simulink model "LQT_Simulation"  (R2015b)
settings: Solver=FixedStepAuto  StartTime=0.0  StopTime=tsim  FixedStep=Ts  RelTol=1e-3
values from neighbouring files (symbols this model uses):
  A_kal = [1 0 0 Ts 0 0 ... (first row only)    [LQT_12states.m]
  C_kal = [1 0 0 0 0 0 ... (first row only)    [LQT_12states.m]
  Ki = [-Ki_coef_ang  -Ki_coef_ang   -Ki_coef_ang ... (first row only)    [LQT_12states.m]
  Ki_LQT = [Ki_coef  -Ki_coef   -Ki_coefz ... (first row only)    [LQT_12states.m]
  R_kal = diag([5e-9 5e-9 5e-9])    [LQT_12states.m]
  Ts = 0.01    [LQT_12states.m]    (also in Trajectory_generation.m)
  VAR_XY = 5e-9    (= 5e-09)    [LQT_12states.m]
  VAR_Z = 5e-9    (= 5e-09)    [LQT_12states.m]
undefined symbols (not defined in the file or in its folder): DiscIntNeverNeededParam, Discrete, pwm, quad, Time
libraries: realtime_pacer_lib x2, ctrlSharedLib x1, aerolibtransform2 x1
settings Model: SimulationMode=accelerator  Creator=carlosluis  LastModifiedBy=carlosluis
settings DebuggingCC: MultiTaskRateTransMsg=warning

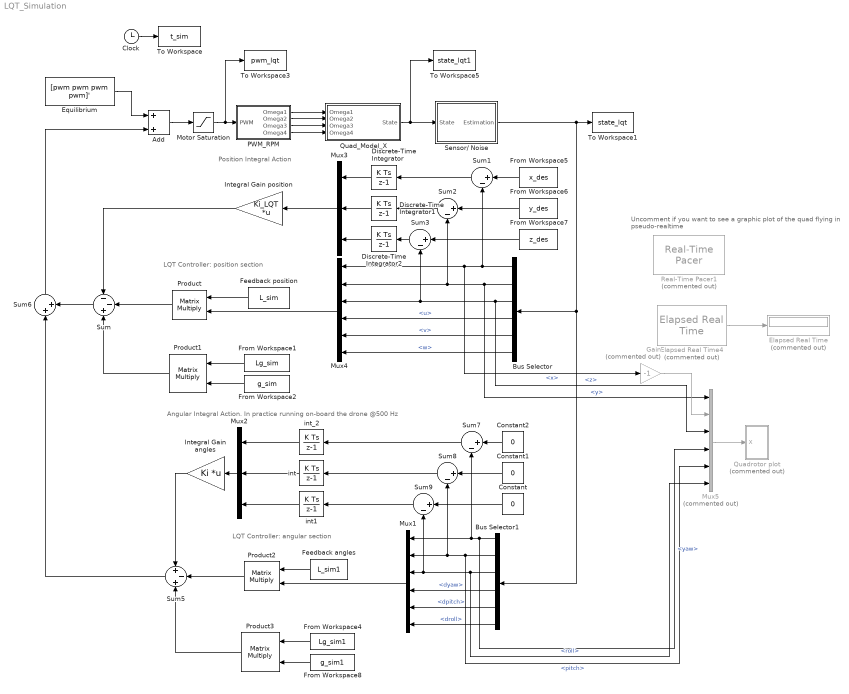
== system LQT_Simulation ==
  note: Uncomment if you want to see a graphic plot of the quad
      | flying in pseudo-realtime
  note: Position Integral Action
  note: Angular Integral Action. In practice running on-board the drone @500 Hz
  note: LQT Controller: position section
  note: LQT Controller: angular section
  Add : Sum
  Bus Selector : BusSelector  OutputSignals=signal1.x,signal1.y,signal1.z,signal3.u,signal3.v,signal3.w
  Bus Selector1 : BusSelector  OutputSignals=signal2.yaw,signal2.pitch,signal2.roll,signal4.dyaw,signal4.dpitch,signal4.droll
  Clock : Clock
  Constant : Constant  Value=0
  Constant1 : Constant  Value=0
  Constant2 : Constant  Value=0
  Discrete-Time Integrator : DiscreteIntegrator  gainval=1  InitialConditionSetting=State (most efficient)  SampleTime=Ts  ICPrevOutput=DiscIntNeverNeededParam  ICPrevScaledInput=DiscIntNeverNeededParam
  Discrete-Time Integrator1 : DiscreteIntegrator  gainval=1  InitialConditionSetting=State (most efficient)  SampleTime=Ts  ICPrevOutput=DiscIntNeverNeededParam  ICPrevScaledInput=DiscIntNeverNeededParam
  Discrete-Time Integrator2 : DiscreteIntegrator  gainval=1  InitialConditionSetting=State (most efficient)  SampleTime=Ts  ICPrevOutput=DiscIntNeverNeededParam  ICPrevScaledInput=DiscIntNeverNeededParam
  Elapsed Real Time : Display  Commented=on
      settings: Decimation=2
  Elapsed Real Time4 : realtime_pacer_lib/Elapsed Real Time  Commented=on
  Equilibrium : Constant  Value=[pwm pwm pwm pwm]'
  Feedback angles : FromWorkspace  VariableName=L_sim1  SampleTime=Ts
  Feedback position : FromWorkspace  VariableName=L_sim  SampleTime=Ts
  From Workspace1 : FromWorkspace  VariableName=Lg_sim  SampleTime=Ts
  From Workspace2 : FromWorkspace  VariableName=g_sim  SampleTime=Ts
  From Workspace4 : FromWorkspace  VariableName=Lg_sim1  SampleTime=Ts
  From Workspace5 : FromWorkspace  VariableName=x_des  SampleTime=Ts
  From Workspace6 : FromWorkspace  VariableName=y_des  SampleTime=Ts
  From Workspace7 : FromWorkspace  VariableName=z_des  SampleTime=Ts
  From Workspace8 : FromWorkspace  VariableName=g_sim1  SampleTime=Ts
  Gain : Gain  Commented=on  Gain=-1
  Integral Gain angles : Gain  Gain=Ki  Multiplication=Matrix(K*u)
  Integral Gain position : Gain  Gain=Ki_LQT  Multiplication=Matrix(K*u)
  Motor Saturation : Saturate  UpperLimit=60000
  Mux1 : Mux  Inputs=6
  Mux2 : Mux  Inputs=3
  Mux3 : Mux  Inputs=3
  Mux4 : Mux  Inputs=6
  Mux5 : Mux  Commented=on  Inputs=6
  PWM_RPM : Subsystem
  Product{,1..3} (4 alike) : Product  Multiplication=Matrix(*)
  Quad_Model_X : Subsystem
  Quadrotor plot : Subsystem  Commented=on  AncestorBlock=roblocks/Robot Graphics/Quadrotor plot  mask{quad=quad, xydim=2, zdim=2.3}
      mask prompts: quad "Model"; xydim "xy-axes dimension"; zdim "z-axis dimension"
      mask help: Animate quadrotor.
      mask Help:
      | This block graphically displays a quadrotor (flying robot).
      | 
      | A new figure is created and A graphical model of a quadrotor is animated
      | to a pose specified by the state vector input to the block.
      | 
      | The state vector is [x y z roll pitch yaw] in world coordinates and the
      | angles are in radians.
      | 
      | Notes:
      | - The dimensions of the vehicle workspace are set by parameters
  Real-Time Pacer1 : realtime_pacer_lib/Real-Time Pacer  Commented=on  simTimePerRealTime=1
  Sensor/ Noise : Subsystem
  Sum : Sum  Inputs=--+
  Sum{1..3,7..9} (6 alike) : Sum  Inputs=|+-
  Sum5 : Sum  Inputs=+-+
  Sum6 : Sum  Inputs=|++
  To Workspace : ToWorkspace  VariableName=t_sim  SampleTime=Ts
  To Workspace1 : ToWorkspace  VariableName=state_lqt  SampleTime=Ts
  To Workspace3 : ToWorkspace  VariableName=pwm_lqt  SampleTime=Ts
  To Workspace5 : ToWorkspace  VariableName=state_lqt1  SampleTime=Ts
  int : DiscreteIntegrator  gainval=1  InitialConditionSetting=State (most efficient)  SampleTime=Ts  ICPrevOutput=DiscIntNeverNeededParam  ICPrevScaledInput=DiscIntNeverNeededParam
  int1 : DiscreteIntegrator  gainval=1  InitialConditionSetting=State (most efficient)  SampleTime=Ts  ICPrevOutput=DiscIntNeverNeededParam  ICPrevScaledInput=DiscIntNeverNeededParam
  int_2 : DiscreteIntegrator  gainval=1  InitialConditionSetting=State (most efficient)  SampleTime=Ts  ICPrevOutput=DiscIntNeverNeededParam  ICPrevScaledInput=DiscIntNeverNeededParam
  wires:
  From Workspace1/1 -> Product1/1
  From Workspace2/1 -> Product1/2
  Feedback position/1 -> Product/1
  Clock/1 -> To Workspace/1
  PWM_RPM/1(Omega1) -> Quad_Model_X/1(Omega1)
  PWM_RPM/2(Omega2) -> Quad_Model_X/2(Omega2)
  PWM_RPM/3(Omega3) -> Quad_Model_X/3(Omega3)
  PWM_RPM/4(Omega4) -> Quad_Model_X/4(Omega4)
  Add/1 -> Motor Saturation/1
  Motor Saturation/1 -> PWM_RPM/1(PWM), To Workspace3/1
  Quad_Model_X/1(State) -> Sensor/ Noise/1(State), To Workspace5/1
  Sensor/ Noise/1(Estimation) -> Bus Selector/1, Bus Selector1/1, To Workspace1/1
  Sum1/1 -> Discrete-Time Integrator/1
  Sum2/1 -> Discrete-Time Integrator1/1
  Sum3/1 -> Discrete-Time Integrator2/1
  Bus Selector1/1 -> Mux5/4, Mux1/1, Sum7/2  "<yaw>"
  Bus Selector1/2 -> Mux5/5, Sum8/2, Mux1/2  "<pitch>"
  Bus Selector1/3 -> Mux5/6, Sum9/2, Mux1/3  "<roll>"
  Bus Selector1/4 -> Mux1/4  "<dyaw>"
  Bus Selector1/5 -> Mux1/5  "<dpitch>"
  Bus Selector1/6 -> Mux1/6  "<droll>"
  From Workspace4/1 -> Product3/1
  From Workspace8/1 -> Product3/2
  Feedback angles/1 -> Product2/1
  Mux1/1 -> Product2/2
  Sum5/1 -> Sum6/1
  int_2/1 -> Mux2/1
  Sum7/1 -> int_2/1
  int/1 -> Mux2/2
  Sum8/1 -> int/1
  Sum9/1 -> int1/1
  int1/1 -> Mux2/3
  Discrete-Time Integrator/1 -> Mux3/1
  Discrete-Time Integrator1/1 -> Mux3/2
  Discrete-Time Integrator2/1 -> Mux3/3
  Mux3/1 -> Integral Gain position/1
  Product3/1 -> Sum5/3
  Product2/1 -> Sum5/2
  Constant/1 -> Sum9/1
  Constant2/1 -> Sum7/1
  Constant1/1 -> Sum8/1
  Mux2/1 -> Integral Gain angles/1
  Integral Gain angles/1 -> Sum5/1
  From Workspace5/1 -> Sum1/1
  From Workspace6/1 -> Sum2/1
  From Workspace7/1 -> Sum3/1
  Bus Selector/1 -> Gain/1, Mux4/1, Sum1/2  "<x>"
  Bus Selector/2 -> Mux5/1, Sum2/2, Mux4/2  "<y>"
  Bus Selector/3 -> Mux5/3, Sum3/2, Mux4/3  "<z>"
  Bus Selector/4 -> Mux4/4  "<u>"
  Bus Selector/5 -> Mux4/5  "<v>"
  Bus Selector/6 -> Mux4/6  "<w>"
  Mux4/1 -> Product/2
  Product1/1 -> Sum/3
  Product/1 -> Sum/2
  Integral Gain position/1 -> Sum/1
  Sum/1 -> Sum6/2
  Sum6/1 -> Add/2
  Equilibrium/1 -> Add/1
  Elapsed Real Time4/1 -> Elapsed Real Time/1
  Mux5/1 -> Quadrotor plot/1(X)
  Gain/1 -> Mux5/2

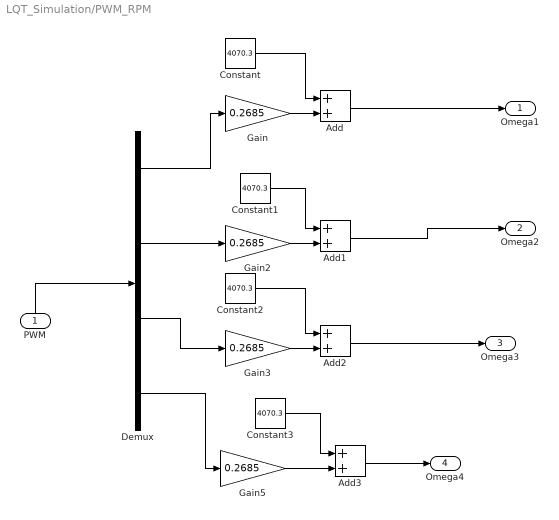
== system LQT_Simulation/PWM_RPM ==
  PWM : Inport
  Add{,1..3} (4 alike) : Sum
  Constant{,1..3} (4 alike) : Constant  Value=4070.3
  Demux : Demux
  Gain{,2..3,5} (4 alike) : Gain  Gain=0.2685
  Omega1 : Outport
  Omega2 : Outport  Port=2
  Omega3 : Outport  Port=3
  Omega4 : Outport  Port=4
  wires:
  Gain/1 -> Add/2
  Demux/1 -> Gain/1
  Demux/4 -> Gain5/1
  Gain5/1 -> Add3/2
  Constant3/1 -> Add3/1
  Add3/1 -> Omega4/1
  Constant1/1 -> Add1/1
  Gain2/1 -> Add1/2
  Demux/2 -> Gain2/1
  Add1/1 -> Omega2/1
  PWM/1 -> Demux/1
  Add/1 -> Omega1/1
  Add2/1 -> Omega3/1
  Demux/3 -> Gain3/1
  Constant2/1 -> Add2/1
  Gain3/1 -> Add2/2
  Constant/1 -> Add/1

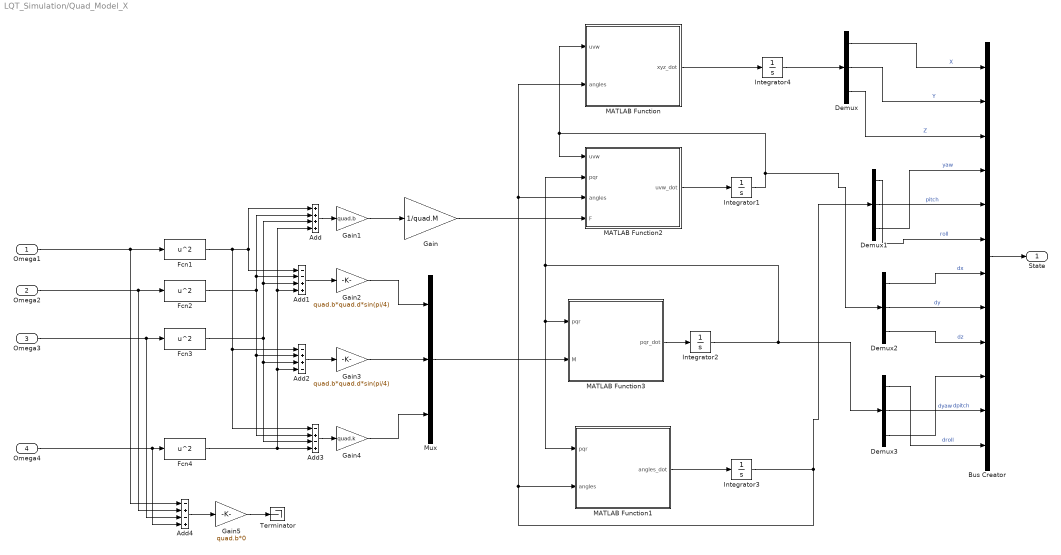
== system LQT_Simulation/Quad_Model_X ==
  Omega1 : Inport
  Omega2 : Inport  Port=2
  Omega3 : Inport  Port=3
  Omega4 : Inport  Port=4
  Add : Sum  Inputs=++++
  Add1 : Sum  Inputs=--++
  Add2 : Sum  Inputs=-++-
  Add3 : Sum  Inputs=-+-+
  Add4 : Sum  Inputs=-+-+
  Bus Creator : BusCreator  Inputs=12
  Demux{,1..3} (4 alike) : Demux  Outputs=3
  Fcn{1..4} (4 alike) : Fcn  Expr=u^2
  Gain : Gain  Gain=1/quad.M
  Gain1 : Gain  Gain=quad.b
  Gain2 : Gain  Gain=quad.b*quad.d*sin(pi/4)
  Gain3 : Gain  Gain=quad.b*quad.d*sin(pi/4)
  Gain4 : Gain  Gain=quad.k
  Gain5 : Gain  Gain=quad.b*0
  Integrator1 : Integrator
  Integrator2 : Integrator
  Integrator3 : Integrator  InitialCondition=[0;0;0]
  Integrator4 : Integrator  InitialCondition=[0;0;0]
  MATLAB Function : MATLAB Function  TreatAsAtomicUnit=on
  MATLAB Function1 : MATLAB Function  TreatAsAtomicUnit=on
  MATLAB Function2 : MATLAB Function  TreatAsAtomicUnit=on
  MATLAB Function3 : MATLAB Function  TreatAsAtomicUnit=on
  Mux : Mux  Inputs=3
  Terminator : Terminator
  State : Outport
  wires:
  Gain1/1 -> Gain/1
  Fcn4/1 -> Add/4, Add1/4, Add2/4, Add3/4
  Fcn3/1 -> Add1/3, Add/3, Add2/3, Add3/3
  Fcn2/1 -> Add2/2, Add3/2, Add1/2, Add/2
  Fcn1/1 -> Add/1, Add1/1, Add2/1, Add3/1
  Bus Creator/1 -> State/1
  Add1/1 -> Gain2/1
  Add/1 -> Gain1/1
  Omega2/1 -> Add4/2, Fcn2/1
  Omega1/1 -> Fcn1/1, Add4/1
  Add2/1 -> Gain3/1
  Gain2/1 -> Mux/1
  Gain4/1 -> Mux/3
  Omega3/1 -> Add4/3, Fcn3/1
  Omega4/1 -> Fcn4/1, Add4/4
  Add4/1 -> Gain5/1
  Add3/1 -> Gain4/1
  Gain3/1 -> Mux/2
  Gain/1 -> MATLAB Function2/4(F)
  Mux/1 -> MATLAB Function3/2(M)
  MATLAB Function2/1(uvw_dot) -> Integrator1/1
  MATLAB Function3/1(pqr_dot) -> Integrator2/1
  MATLAB Function1/1(angles_dot) -> Integrator3/1
  Integrator1/1 -> MATLAB Function/1(uvw), MATLAB Function2/1(uvw), Demux2/1
  Integrator2/1 -> Demux3/1, MATLAB Function2/2(pqr), MATLAB Function1/1(pqr), MATLAB Function3/1(pqr)
  Demux/1 -> Bus Creator/1  "X"
  Demux/2 -> Bus Creator/2  "Y"
  Demux/3 -> Bus Creator/3  "Z"
  Demux1/3 -> Bus Creator/4  "yaw"
  Demux1/1 -> Bus Creator/6  "roll"
  Demux2/1 -> Bus Creator/7  "dx"
  Demux2/2 -> Bus Creator/8  "dy"
  Demux2/3 -> Bus Creator/9  "dz"
  Demux3/3 -> Bus Creator/10  "dyaw"
  Demux3/2 -> Bus Creator/11  "dpitch"
  Demux3/1 -> Bus Creator/12  "droll"
  Gain5/1 -> Terminator/1
  Demux1/2 -> Bus Creator/5  "pitch"
  Integrator3/1 -> Demux1/1, MATLAB Function/2(angles), MATLAB Function2/3(angles), MATLAB Function1/2(angles)
  MATLAB Function/1(xyz_dot) -> Integrator4/1
  Integrator4/1 -> Demux/1

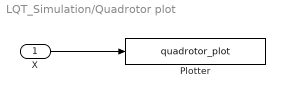
== system LQT_Simulation/Quadrotor plot ==
  X : Inport
  Plotter : S-Function  FunctionName=quadrotor_plot  Parameters=[xydim, zdim], 1, 1,quad  SFunctionDeploymentMode=off  EnableBusSupport=off
  wires:
  X/1 -> Plotter/1

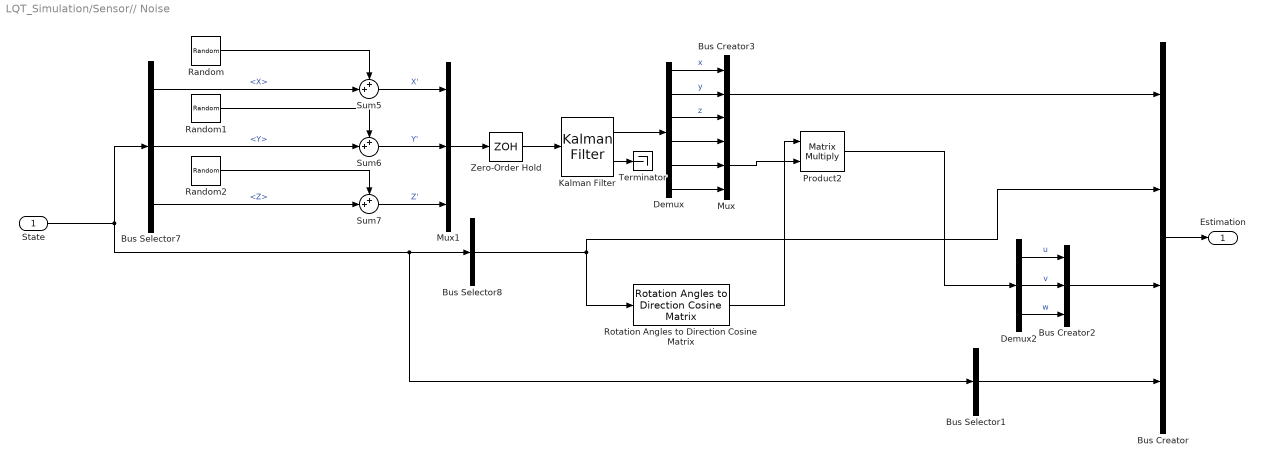
== system LQT_Simulation/Sensor// Noise ==
  State : Inport
  Bus Creator : BusCreator  Inputs=4
  Bus Creator2 : BusCreator  Inputs=3
  Bus Creator3 : BusCreator  Inputs=3
  Bus Selector1 : BusSelector  OutputSignals=dyaw,dpitch,droll  OutputAsBus=on
  Bus Selector7 : BusSelector  OutputSignals=X,Y,Z
  Bus Selector8 : BusSelector  OutputSignals=yaw,pitch,roll  OutputAsBus=on
  Demux : Demux  Outputs=6
  Demux2 : Demux  Outputs=3
  Kalman Filter : ctrlSharedLib/Kalman Filter  TimeDomain=Discrete-Time  UseCurrentEstimator=on  ModelSource=Individual A, B, C, D matrices  ModelSourceVariable=ss(0.95,1,1,0,1)  A=A_kal  B=1  C=C_kal  D=0  NumberOfStates=1  NumberOfInputs=1  NumberOfOutputs=1  InitialEstimateSource=Dialog  X0=0  P0=10  UseK=off  UseGH=on  NumberOfProcessNoiseInputs=1  G=G_kal  TimeInvariantG=on  H=0  TimeInvariantH=on  Q=Q_kal  TimeInvariantQ=on  R=R_kal  TimeInvariantR=on  N=0  TimeInvariantN=on  AddInputPort=off  AddEnablePort=off  OutputEstimatedY=off  OutputP=on  Ts=Ts
  Mux : Mux  Inputs=3
  Mux1 : Mux  Inputs=3
  Product2 : Product  Multiplication=Matrix(*)
  Random : RandomNumber  Variance=VAR_XY  SampleTime=Ts
  Random1 : RandomNumber  Variance=VAR_XY  SampleTime=Ts
  Random2 : RandomNumber  Variance=VAR_Z  SampleTime=Ts
  Rotation Angles to Direction Cosine Matrix : aerolibtransform2/Rotation Angles to Direction Cosine Matrix  rotationOrder=ZYX
  Sum5 : Sum  Inputs=++|
  Sum6 : Sum  Inputs=++|
  Sum7 : Sum  Inputs=++|
  Terminator : Terminator
  Zero-Order Hold : ZeroOrderHold  SampleTime=Ts
  Estimation : Outport
  wires:
  Bus Selector8/1 -> Bus Creator/2, Rotation Angles to Direction Cosine Matrix/1
  Product2/1 -> Demux2/1
  Rotation Angles to Direction Cosine Matrix/1 -> Product2/1
  Kalman Filter/1 -> Demux/1
  Zero-Order Hold/1 -> Kalman Filter/1
  Mux1/1 -> Zero-Order Hold/1
  Bus Creator3/1 -> Bus Creator/1
  Demux/3 -> Bus Creator3/3  "z"
  Demux/2 -> Bus Creator3/2  "y"
  Demux/1 -> Bus Creator3/1  "x"
  Mux/1 -> Product2/2
  Demux/4 -> Mux/1
  Demux/5 -> Mux/2
  Demux/6 -> Mux/3
  Bus Creator2/1 -> Bus Creator/3
  Bus Selector1/1 -> Bus Creator/4
  Demux2/3 -> Bus Creator2/3  "w"
  Demux2/2 -> Bus Creator2/2  "v"
  Demux2/1 -> Bus Creator2/1  "u"
  Random2/1 -> Sum7/1
  Sum7/1 -> Mux1/3  "Z'"
  Sum6/1 -> Mux1/2  "Y'"
  Sum5/1 -> Mux1/1  "X'"
  Bus Selector7/3 -> Sum7/2  "<Z>"
  Bus Selector7/2 -> Sum6/2  "<Y>"
  Bus Selector7/1 -> Sum5/2  "<X>"
  Bus Creator/1 -> Estimation/1
  State/1 -> Bus Selector7/1, Bus Selector1/1, Bus Selector8/1
  Random1/1 -> Sum6/1
  Random/1 -> Sum5/1
  Kalman Filter/2 -> Terminator/1

== matlab function LQT_Simulation/Quad_Model_X/MATLAB Function ==
  data: uvw input; xyz_dot output; angles input
function xyz_dot  = Position(uvw,angles)
xyz_dot = zeros(3,1);
phi = angles(1); %*pi/180;
theta = angles(2); %*pi/180;
psi = angles(3); %*pi/180;
Tb_o = [cos(theta)*cos(psi)                                cos(theta)*sin(psi)                             -sin(theta)  ;   %BBF > Inertial rotation matrix
        sin(phi)*sin(theta)*cos(psi)-cos(phi)*sin(psi)    sin(phi)*sin(theta)*sin(psi)+cos(phi)*cos(psi)  sin(phi)*cos(theta) ;
        cos(phi)*sin(theta)*cos(psi)+sin(phi)*sin(psi)    cos(phi)*sin(theta)*sin(psi)-sin(phi)*cos(psi)   cos(phi)*cos(theta)];

xyz_dot = (Tb_o')*uvw;
end

== matlab function LQT_Simulation/Quad_Model_X/MATLAB Function1 ==
  data: pqr input; angles_dot output; angles input
function angles_dot  = Angle(pqr,angles)
angles_dot = zeros(3,1);
phi = angles(1); %*pi/180;
theta = angles(2); %*pi/180;

H = [1    sin(phi)*tan(theta)     cos(phi)*tan(theta)
     0       cos(phi)                 -sin(phi)   
     0       sin(phi)/cos(theta)    cos(phi)/cos(theta)];
angles_dot = H*pqr;
end

== matlab function LQT_Simulation/Quad_Model_X/MATLAB Function2 ==
  data: uvw input; uvw_dot output; pqr input; angles input; F input
function uvw_dot  = Forces(uvw,pqr,angles,F)
uvw_dot = zeros(3,1);
Force = [0;0;F];
g_o = [0;0;-9.81];
phi = angles(1); %*pi/180;
theta = angles(2); %*pi/180;
psi = angles(3); %*pi/180;
Tb_o = [cos(theta)*cos(psi)                                cos(theta)*sin(psi)                             -sin(theta)  ;   %BBF > Inertial rotation matrix
        sin(phi)*sin(theta)*cos(psi)-cos(phi)*sin(psi)    sin(phi)*sin(theta)*sin(psi)+cos(phi)*cos(psi)  sin(phi)*cos(theta) ;
        cos(phi)*sin(theta)*cos(psi)+sin(phi)*sin(psi)    cos(phi)*sin(theta)*sin(psi)-sin(phi)*cos(psi)   cos(phi)*cos(theta)];

uvw_dot = Force + Tb_o*g_o - cross(pqr,uvw);

end

== matlab function LQT_Simulation/Quad_Model_X/MATLAB Function3 ==
  data: pqr_dot output; pqr input; M input
function pqr_dot  = Moments(pqr,M)
pqr_dot = zeros(3,1);
Ixx =  1.395e-05;  %2.3951e-5; %1.39e-05; %2.51943e-5; % % %
Iyy = 1.436e-05; %2.3951e-5; %1.436e-05; % 2.54379e-5; % %         %
Izz =  2.173e-05;  %3.2347e-5; %2.173e-05 ; %4.51407e-5; % %         %;%0.160;
J = diag([Ixx Iyy Izz]);    %   I  Flyer rotational inertia matrix     3x3
pqr_dot = inv(J)*(M-cross(pqr,J*pqr));
end
